simulink model "Weak_magnetic"  (R2014a)
settings: Solver=ode15s  StartTime=0.0  StopTime=50  RelTol=1e-3
libraries: powerlib x19, powerlib_meascontrol x1
settings Model: Creator=lenovo  LastModifiedBy=DELL
settings SolverCC: ZeroCrossAlgorithm=Adaptive
settings DebuggingCC: MergeDetectMultiDrivingBlocksExec=error  FrameProcessingCompatibilityMsg=error
settings SimscapeCC: SimscapeNormalizeSystem=off
settings ConfigurationSet: Description=Simscape Multibody

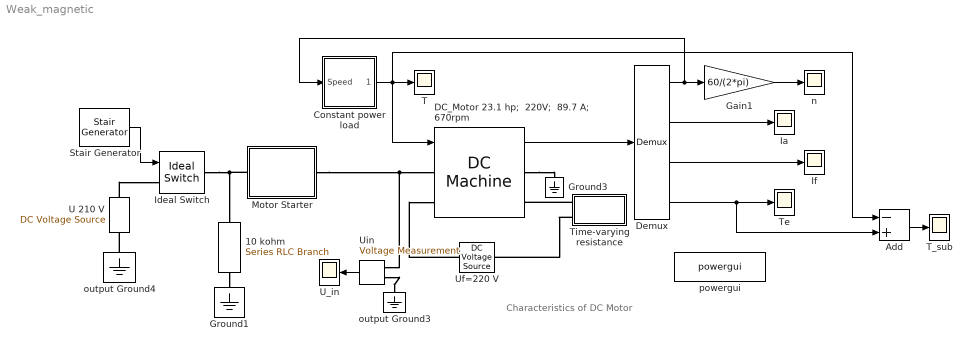
== system Weak_magnetic ==
  note: Characteristics of DC Motor
  10 kohm : powerlib/Elements/Series RLC Branch  LConnTagsString=__new0  RConnTagsString=__new0  BranchType=R  Resistance=1e4  Inductance=[]  SetiL0=off  InitialCurrent=0  Capacitance=[]  Setx0=off  InitialVoltage=0  Measurements=None
  Add : Sum  Inputs=-+
  Constant power load : Subsystem
  DC_Motor 23.1 hp;  220V;  89.7 A;  670rpm : powerlib/Machines/DC Machine  PresetModel=No  MechanicalLoad=Torque TL  FieldType=Wound  ShowDetailedParameters=on  MeasurementBus=off  RLa="[ 0.2  0.0140]"  RLf="[ 183.333  0]"  Laf=2.400  MachineConstant=Torque constant (N.m/A)  Ke=1.8  Kt=1.8  J=0.76  Bm=0  Tf=16.055  w0=1  Ifinit=1  TsPowergui=0  TsBlock=-1
      settings: AttributesFormatString=\n
  Demux : Demux
      settings: DisplayOption=none
  Gain1 : Gain  Gain=60/(2*pi)
  Ground1 : powerlib/Elements/Ground  LConnTagsString=a
  Ground3 : powerlib/Elements/Ground  LConnTagsString=a
  Ia : Scope
      settings: TimeRange=10  TickLabels=on  MaxDataPoints=500000  SaveName=Ia  YMin=0  YMax=40  SampleInput=on  SampleTime=0.01  DataFormat=Array
  Ideal Switch : powerlib/Power Electronics/Ideal Switch  Ron=1e-4  Lon=10e-6  IC=0  Rs=inf  Cs=0  Measurements=off
      settings: AttributesFormatString=\n
  If : Scope
      settings: TimeRange=10  TickLabels=on  MaxDataPoints=500000  SaveName=lf  YMin=0  YMax=40  SampleInput=on  SampleTime=0.01  DataFormat=Array
  Motor Starter : Subsystem
      mask Display: disp('3 step\n\nstarter')
  Stair Generator : powerlib_meascontrol/Pulse & Signal Generators/Stair Generator  t=[0 0.5 ]  e=[0 1 ]  Ts=0
  T : Scope
      settings: TimeRange=10  TickLabels=on  MaxDataPoints=500000  SaveName=T  YMin=-35.24494  YMax=317.20449  SampleInput=on  SampleTime=0.01  DataFormat=Array
  T_sub : Scope
      settings: TimeRange=10  TickLabels=on  MaxDataPoints=500000  SaveName=Te1  YMin=-25.91438  YMax=83.64158  SampleInput=on  SampleTime=0.01  DataFormat=Array
  Te : Scope
      settings: TimeRange=10  TickLabels=on  MaxDataPoints=500000  SaveName=Te  YMin=-38.71026  YMax=348.38581  SampleInput=on  SampleTime=0.01  DataFormat=Array
  Time-varying resistance : Subsystem
  U 210 V : powerlib/Electrical Sources/DC Voltage Source  Description=source block  Amplitude=200  Measurements=None
      settings: AttributesFormatString=\n
  U_in : Scope
      settings: TimeRange=10  TickLabels=on  MaxDataPoints=500000  SaveName=U_in  YMin=-24.99289  YMax=224.933  SampleInput=on  SampleTime=0.01  DataFormat=Array
  Uf=220 V : powerlib/Electrical Sources/DC Voltage Source  Description=source block  Amplitude=220  Measurements=None
      settings: AttributesFormatString=\n
  Uin : powerlib/Measurements/Voltage Measurement  Tag=PoWeRsYsTeMmEaSuReMeNt  PhasorSimulation=off  OutputType=Magnitude  PSBequivalent=0
  n : Scope
      settings: TimeRange=10  TickLabels=on  MaxDataPoints=500000  SaveName=n  YMin=-96.84018  YMax=871.54898  SampleInput=on  SampleTime=0.01  DataFormat=Array
  output Ground3 : powerlib/Elements/Ground  LConnTagsString=a
  output Ground4 : powerlib/Elements/Ground  LConnTagsString=a
  powergui : powerlib/powergui  Priority=2  SimulationMode=Continuous  SampleTime=0  frequency=60  Iterations=50  frequencyindice=0  Pbase=100e6  ErrMax=1e-4  UnitsV=kV  UnitsW=MW  buscounter=0  FunctionMessages=off  echomessages=off  EnableUseOfTLC=off  CurrentSourceSwitches=off  DisableSnubberDevices=off  DisableRonSwitches=off  DisableVfSwitches=off  DisplayEquations=off  AutomaticDiscreteSolvers=off  SolverType=Tustin  Interpol=off  ExternalGateDelay=off  methode=off  Ts=0  x0status=blocks  SPID=off  SwTol=0  HookPort=off  NonlinearTolerance=1e-4  nMaxIteration=100  ContinueOnMaxIteration=off  RestoreLinks=warning  ResistiveCurrentMeasurement=off  Frange=logspace(0,3,50)  Ylog=off  Xlog=off  ShowGrid=off  save=off  variable=ZData  structure=0  ZoomFFT=on  StartTime=0.0  cycles=1  DisplayStyle=off  fundamental=60  FreqAxis=off  MaxFrequency=1000  frequencyindicesteady=1  RmsSteady=1  display=off
  wires:
  Stair Generator/1 -> Ideal Switch/1
  Gain1/1 -> n/1
  DC_Motor 23.1 hp;  220V;  89.7 A;  670rpm/1 -> Demux/1
  Demux/1 -> Gain1/1, Constant power load/1(Speed)
  Demux/2 -> Ia/1
  Demux/4 -> Add/2, Te/1
  Uin/1 -> U_in/1
  Constant power load/1(" ") -> T/1, Add/1, DC_Motor 23.1 hp;  220V;  89.7 A;  670rpm/1
  Demux/3 -> If/1
  Add/1 -> T_sub/1
  connections:
  Ideal Switch/RConn1 -- 10 kohm/LConn1 -- Motor Starter/LConn1
  U 210 V/RConn1 -- Ideal Switch/LConn1
  DC_Motor 23.1 hp;  220V;  89.7 A;  670rpm/RConn1 -- Ground3/LConn1
  output Ground4/LConn1 -- U 210 V/LConn1
  Uf=220 V/RConn1 -- DC_Motor 23.1 hp;  220V;  89.7 A;  670rpm/LConn2
  10 kohm/RConn1 -- Ground1/LConn1
  Uin/LConn1 -- Motor Starter/RConn1 -- DC_Motor 23.1 hp;  220V;  89.7 A;  670rpm/LConn1
  Uin/LConn2 -- output Ground3/LConn1
  Time-varying resistance/LConn1 -- DC_Motor 23.1 hp;  220V;  89.7 A;  670rpm/RConn2
  Time-varying resistance/LConn2 -- Uf=220 V/LConn1

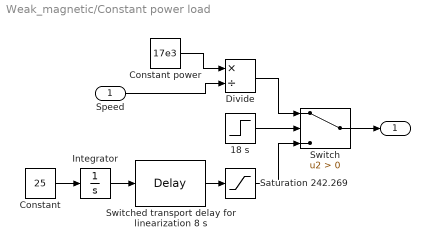
== system Weak_magnetic/Constant power load ==
  Speed : Inport
  18 s : Step  Time=18  Before=-1  SampleTime=0
  Constant : Constant  Value=25
  Constant power : Constant  Value=17e3
  Divide : Product  Inputs=*/
  Integrator : Integrator
  Saturation 242.269 : Saturate  UpperLimit=242.269  LowerLimit=0
  Switch : Switch  Criteria=u2 > Threshold
  Switched transport delay for linearization 8 s : TransportDelay  DelayTime=8  PadeOrder=2
  " " : Outport
  wires:
  Constant/1 -> Integrator/1
  Switched transport delay for linearization 8 s/1 -> Saturation 242.269/1
  Integrator/1 -> Switched transport delay for linearization 8 s/1
  Constant power/1 -> Divide/1
  Switch/1 -> " "/1
  Saturation 242.269/1 -> Switch/3
  Divide/1 -> Switch/1
  18 s/1 -> Switch/2
  Speed/1 -> Divide/2

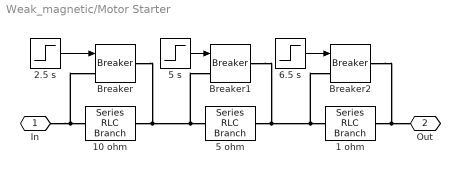
== system Weak_magnetic/Motor Starter ==
  1 ohm : powerlib/Elements/Series RLC Branch  LConnTagsString=__new0  RConnTagsString=__new0  BranchType=R  Resistance=1  Inductance=[]  SetiL0=off  InitialCurrent=0  Capacitance=[]  Setx0=off  InitialVoltage=0  Measurements=None
  10 ohm : powerlib/Elements/Series RLC Branch  LConnTagsString=__new0  RConnTagsString=__new0  BranchType=R  Resistance=10  Inductance=[]  SetiL0=off  InitialCurrent=0  Capacitance=[]  Setx0=off  InitialVoltage=0  Measurements=None
  2.5 s : Step  Time=2.5  SampleTime=0
  5 ohm : powerlib/Elements/Series RLC Branch  LConnTagsString=__new0  RConnTagsString=__new0  BranchType=R  Resistance=5  Inductance=[]  SetiL0=off  InitialCurrent=0  Capacitance=[]  Setx0=off  InitialVoltage=0  Measurements=None
  5 s : Step  Time=5  SampleTime=0
  6.5 s : Step  Time=6.5  SampleTime=0
  Breaker : powerlib/Elements/Breaker  InitialState=0  SwitchingTimes="[ 4/60  5/60 ]"  External=on  BreakerResistance=0.01  SnubberResistance=inf  SnubberCapacitance=0  Measurements=None  MoreParameters=off  NoBreakLoop=off
      settings: AttributesFormatString=\n
  Breaker1 : powerlib/Elements/Breaker  InitialState=0  SwitchingTimes="[ 4/60  5/60 ]"  External=on  BreakerResistance=0.01  SnubberResistance=inf  SnubberCapacitance=0  Measurements=None  MoreParameters=off  NoBreakLoop=off
      settings: AttributesFormatString=\n
  Breaker2 : powerlib/Elements/Breaker  InitialState=0  SwitchingTimes="[ 4/60  5/60 ]"  External=on  BreakerResistance=0.01  SnubberResistance=inf  SnubberCapacitance=0  Measurements=None  MoreParameters=off  NoBreakLoop=off
      settings: AttributesFormatString=\n
  In : PMIOPort  Side=Left
  Out : PMIOPort  Port=2  Side=Right
  wires:
  5 s/1 -> Breaker1/1
  6.5 s/1 -> Breaker2/1
  2.5 s/1 -> Breaker/1
  connections:
  In/RConn1 -- 10 ohm/LConn1 -- Breaker/LConn1
  10 ohm/RConn1 -- Breaker/RConn1 -- 5 ohm/LConn1 -- Breaker1/LConn1
  5 ohm/RConn1 -- Breaker1/RConn1 -- 1 ohm/LConn1 -- Breaker2/LConn1
  1 ohm/RConn1 -- Breaker2/RConn1 -- Out/RConn1

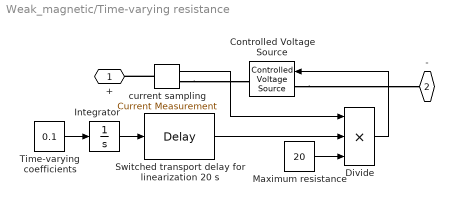
== system Weak_magnetic/Time-varying resistance ==
  Controlled Voltage Source : powerlib/Electrical Sources/Controlled Voltage Source  Initialize=on  Source_Type=AC  Amplitude=0  Phase=0  Frequency=0  Measurements=None
  Divide : Product  Inputs=***
  Integrator : Integrator
  Maximum resistance : Constant  Value=20
  Switched transport delay for linearization 20 s : TransportDelay  DelayTime=20  PadeOrder=2
  Time-varying coefficients : Constant  Value=0.1
  current sampling : powerlib/Measurements/Current Measurement  PhasorSimulation=off  OutputType=Complex  PSBequivalent=0
  + : PMIOPort  Side=Left
  - : PMIOPort  Port=2  Side=Left
  wires:
  Divide/1 -> Controlled Voltage Source/1
  current sampling/1 -> Divide/1
  Time-varying coefficients/1 -> Integrator/1
  Maximum resistance/1 -> Divide/3
  Switched transport delay for linearization 20 s/1 -> Divide/2
  Integrator/1 -> Switched transport delay for linearization 20 s/1
  connections:
  current sampling/RConn1 -- Controlled Voltage Source/RConn1
  current sampling/LConn1 -- +/RConn1
  Controlled Voltage Source/LConn1 -- -/RConn1
